simulink model "kiok"  (Simulink 4.00)
settings: Solver=ode45  StartTime=0.0  StopTime=10.0  RelTol=1e-3
settings Model: LastModifiedBy=user

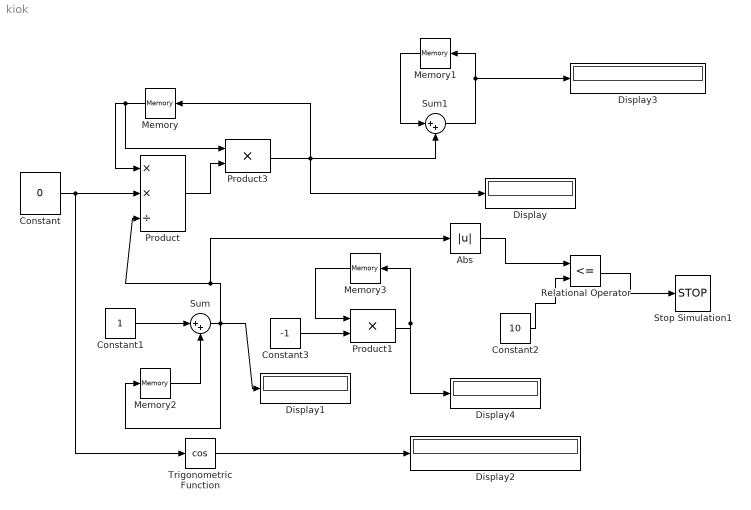
== system kiok ==
  Abs : Abs  SaturateOnIntegerOverflow=on
  Constant : Constant  Value=0
  Constant1 : Constant  Value=1
  Constant2 : Constant  Value=10
  Constant3 : Constant  Value=-1
  Display{,1..4} (5 alike) : Display
      Display settings: Format=short
      Display1 settings: Format=short
      Display4 settings: Format=short
  Memory : Memory  Orientation=left  X0=1  InheritSampleTime=off
      settings: RTWStateStorageClass=Auto
  Memory1 : Memory  Orientation=left  X0=1  InheritSampleTime=off
      settings: RTWStateStorageClass=Auto
  Memory2 : Memory  X0=0  InheritSampleTime=off
      settings: RTWStateStorageClass=Auto
  Memory3 : Memory  Orientation=left  X0=1  InheritSampleTime=off
      settings: RTWStateStorageClass=Auto
  Product : Product  Inputs=**/  Multiplication=Element-wise(.*)  SaturateOnIntegerOverflow=on
  Product1 : Product  Inputs=2  Multiplication=Element-wise(.*)  SaturateOnIntegerOverflow=on
  Product3 : Product  Inputs=2  Multiplication=Element-wise(.*)  SaturateOnIntegerOverflow=on
  Relational Operator : RelationalOperator  Operator=<=
  Stop Simulation1 : Stop
  Sum : Sum  Inputs=|++  SaturateOnIntegerOverflow=on
  Sum1 : Sum  Inputs=|++  SaturateOnIntegerOverflow=on
  Trigonometric Function : Trigonometry  Operator=cos  OutputSignalType=auto
  wires:
  Constant/1 -> Product/2, Trigonometric Function/1
  Trigonometric Function/1 -> Display2/1
  Constant1/1 -> Sum/1
  Memory2/1 -> Sum/2
  Memory/1 -> Product/1, Product3/1
  Memory1/1 -> Sum1/1
  Sum1/1 -> Memory1/1, Display3/1
  Sum/1 -> Memory2/1, Display1/1, Product/3, Abs/1
  Abs/1 -> Relational Operator/1
  Constant2/1 -> Relational Operator/2
  Relational Operator/1 -> Stop Simulation1/1
  Constant3/1 -> Product1/2
  Memory3/1 -> Product1/1
  Product1/1 -> Memory3/1, Display4/1
  Product/1 -> Product3/2
  Product3/1 -> Memory/1, Sum1/2, Display/1
